simulink model "min_cost_function_and_vopt_FCS_MPC_6Phase_PMSM"  (R2022a)
settings: Solver=FixedStepDiscrete  StartTime=0.0  StopTime=10.0  RelTol=1e-3
values from neighbouring files (symbols this model uses):
  f_c = 100000    [MPC_params.m]
libraries: hdlsllib x2
settings Model: DataTypeOverride=Off  Creator=Andre Merx  LastModifiedBy=Andre Merx
settings SolverCC: AlgebraicLoopSolver=TrustRegion
settings DataIOCC: LimitDataPoints=on  SaveOutput=off  SaveTime=off
settings OptimizationCC: BlockReduction=off  ConditionallyExecuteInputs=off  DefaultParameterBehavior=Inlined  LifeSpan=inf
settings DebuggingCC: AlgebraicLoopMsg=error  SingleTaskRateTransMsg=error  UnconnectedInputMsg=warning  UnconnectedOutputMsg=warning  UnconnectedLineMsg=warning  AllowSymbolicDim=off  StrictBusMsg=ErrorOnBusTreatedAsVector  SFUnexpectedBacktrackingDiag=warning  SFNoUnconditionalDefaultTransitionDiag=warning  SFExecutionAtInitializationDiag=none  SFMachineParentedDataDiag=warning  ArithmeticOperatorsInVariantConditions=warning
settings HardwareCC: ProdBitPerPointer=32  ProdBitPerSizeT=32  ProdBitPerPtrDiffT=32  ProdLargestAtomicFloat=None  ProdIntDivRoundTo=Undefined  ProdEndianess=Unspecified  ProdWordSize=32  ProdHWDeviceType=ASIC/FPGA->ASIC/FPGA  ProdEqTarget=off
settings SFSimCC: SimUseLocalCustomCode=off  CustomCodeUndefinedFunction=UseInterfaceOnly
settings RTWCC: RTWUseLocalCustomCode=off
settings CodeAppCC: StateflowObjectComments=on
settings GRTTargetCC: TargetLangStandard=C89/C90 (ANSI)
settings ConfigComp: CovScope=ReferencedModels  CovMetricSettings=dw  CovSaveCumulativeToWorkspaceVar=on  CovSaveSingleToWorkspaceVar=on  CovExternalEMLEnable=off  CovSFcnEnable=off

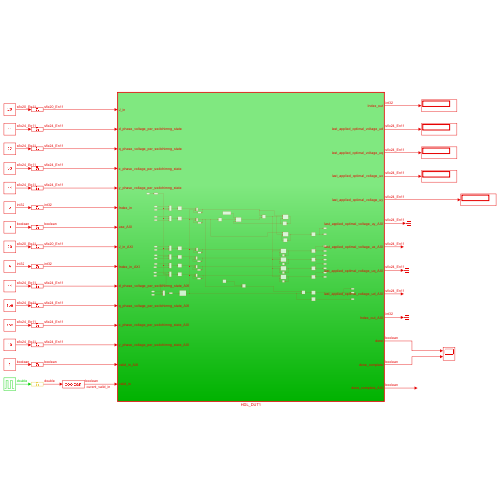
[thumbnail: Simulink's stored preview of the top-level diagram]
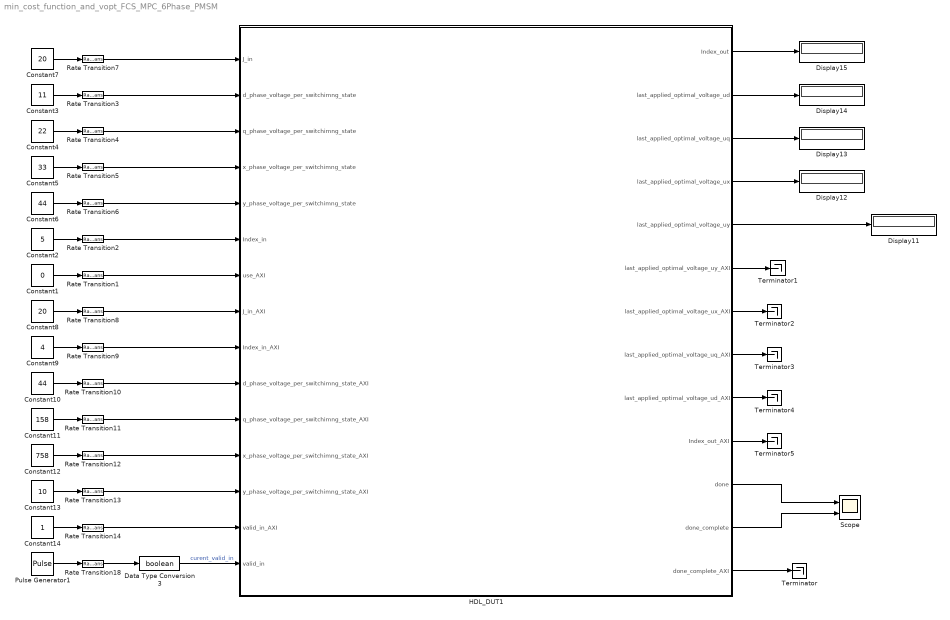
== system min_cost_function_and_vopt_FCS_MPC_6Phase_PMSM ==
  Constant1 : Constant  Value=0  OutDataTypeStr=boolean  SampleTime=-1
  Constant10 : Constant  Value=44  OutDataTypeStr=fixdt(1,24,11)  SampleTime=-1  LockScale=on
  Constant11 : Constant  Value=158  OutDataTypeStr=fixdt(1,24,11)  SampleTime=-1
  Constant12 : Constant  Value=758  OutDataTypeStr=fixdt(1,24,11)  SampleTime=-1
  Constant13 : Constant  Value=10  OutDataTypeStr=fixdt(1,24,11)  SampleTime=-1
  Constant14 : Constant  OutDataTypeStr=boolean  SampleTime=-1
  Constant2 : Constant  Value=5  OutDataTypeStr=int32  SampleTime=-1
  Constant3 : Constant  Value=11  OutDataTypeStr=fixdt(1,24,11)  SampleTime=-1  LockScale=on
  Constant4 : Constant  Value=22  OutDataTypeStr=fixdt(1,24,11)  SampleTime=-1
  Constant5 : Constant  Value=33  OutDataTypeStr=fixdt(1,24,11)  SampleTime=-1
  Constant6 : Constant  Value=44  OutDataTypeStr=fixdt(1,24,11)  SampleTime=-1
  Constant7 : Constant  Value=20  OutDataTypeStr=fixdt(1,20,11)  SampleTime=-1
  Constant8 : Constant  Value=20  OutDataTypeStr=fixdt(1,20,11)  SampleTime=-1
  Constant9 : Constant  Value=4  OutDataTypeStr=int32  SampleTime=-1
  Data Type Conversion3 : DataTypeConversion  OutDataTypeStr=boolean  SaturateOnIntegerOverflow=off  RndMeth=Floor
  Display{11..15} (5 alike) : Display
  HDL_DUT1 : Subsystem  TreatAsAtomicUnit=on
  Pulse Generator1 : DiscretePulseGenerator  PulseType=Time based  Period=1/f_c
  Rate Transition{1..14,18} (15 alike) : RateTransition  OutPortSampleTime=Rt
  Scope : Scope  NumInputPorts=2
  Terminator{,1..5} (6 alike) : Terminator
  wires:
  Data Type Conversion3/1 -> HDL_DUT1/15(valid_in)  "curent_valid_in"
  Pulse Generator1/1 -> Rate Transition18/1
  Rate Transition18/1 -> Data Type Conversion3/1
  Constant2/1 -> Rate Transition2/1
  Rate Transition2/1 -> HDL_DUT1/6(Index_in)
  HDL_DUT1/5(last_applied_optimal_voltage_uy) -> Display11/1
  HDL_DUT1/4(last_applied_optimal_voltage_ux) -> Display12/1
  HDL_DUT1/3(last_applied_optimal_voltage_uq) -> Display13/1
  HDL_DUT1/2(last_applied_optimal_voltage_ud) -> Display14/1
  HDL_DUT1/1(Index_out) -> Display15/1
  Constant3/1 -> Rate Transition3/1
  Rate Transition3/1 -> HDL_DUT1/2(d_phase_voltage_per_switchimng_state)
  Constant4/1 -> Rate Transition4/1
  Rate Transition4/1 -> HDL_DUT1/3(q_phase_voltage_per_switchimng_state)
  Constant5/1 -> Rate Transition5/1
  Rate Transition5/1 -> HDL_DUT1/4(x_phase_voltage_per_switchimng_state)
  Constant6/1 -> Rate Transition6/1
  Rate Transition6/1 -> HDL_DUT1/5(y_phase_voltage_per_switchimng_state)
  Constant7/1 -> Rate Transition7/1
  Rate Transition7/1 -> HDL_DUT1/1(J_in)
  HDL_DUT1/13(done_complete_AXI) -> Terminator/1
  HDL_DUT1/6(last_applied_optimal_voltage_uy_AXI) -> Terminator1/1
  HDL_DUT1/7(last_applied_optimal_voltage_ux_AXI) -> Terminator2/1
  HDL_DUT1/8(last_applied_optimal_voltage_uq_AXI) -> Terminator3/1
  HDL_DUT1/9(last_applied_optimal_voltage_ud_AXI) -> Terminator4/1
  HDL_DUT1/10(Index_out_AXI) -> Terminator5/1
  Constant1/1 -> Rate Transition1/1
  Rate Transition1/1 -> HDL_DUT1/7(use_AXI)
  Constant8/1 -> Rate Transition8/1
  Rate Transition8/1 -> HDL_DUT1/8(J_in_AXI)
  Constant9/1 -> Rate Transition9/1
  Rate Transition9/1 -> HDL_DUT1/9(Index_in_AXI)
  Rate Transition12/1 -> HDL_DUT1/12(x_phase_voltage_per_switchimng_state_AXI)
  Constant11/1 -> Rate Transition11/1
  Constant12/1 -> Rate Transition12/1
  Constant13/1 -> Rate Transition13/1
  Rate Transition13/1 -> HDL_DUT1/13(y_phase_voltage_per_switchimng_state_AXI)
  Constant10/1 -> Rate Transition10/1
  Rate Transition11/1 -> HDL_DUT1/11(q_phase_voltage_per_switchimng_state_AXI)
  Rate Transition10/1 -> HDL_DUT1/10(d_phase_voltage_per_switchimng_state_AXI)
  Constant14/1 -> Rate Transition14/1
  Rate Transition14/1 -> HDL_DUT1/14(valid_in_AXI)
  HDL_DUT1/11(done) -> Scope/1
  HDL_DUT1/12(done_complete) -> Scope/2

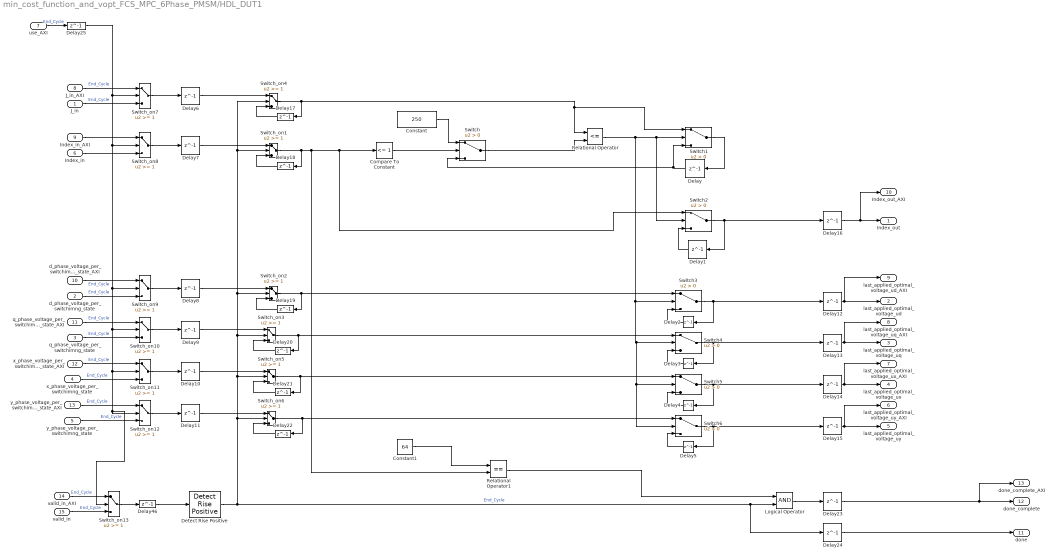
== system min_cost_function_and_vopt_FCS_MPC_6Phase_PMSM/HDL_DUT1 ==
  J_in : Inport
  d_phase_voltage_per_switchimng_state : Inport  Port=2
  q_phase_voltage_per_switchimng_state : Inport  Port=3
  x_phase_voltage_per_switchimng_state : Inport  Port=4
  y_phase_voltage_per_switchimng_state : Inport  Port=5
  Index_in : Inport  Port=6
  use_AXI : Inport  Port=7
  J_in_AXI : Inport  Port=8
  Index_in_AXI : Inport  Port=9
  d_phase_voltage_per_switchimng_state_AXI : Inport  Port=10
  q_phase_voltage_per_switchimng_state_AXI : Inport  Port=11
  x_phase_voltage_per_switchimng_state_AXI : Inport  Port=12
  y_phase_voltage_per_switchimng_state_AXI : Inport  Port=13
  valid_in_AXI : Inport  Port=14
  valid_in : Inport  Port=15
  Compare To Constant : hdlsllib/Logic and Bit Operations/Compare To Constant  relop=<=  const=1  OutDataTypeStr=boolean
      settings: SourceProductBaseCode=SL
  Constant : Constant  Value=250  OutDataTypeStr=fixdt(1,20,11)  SampleTime=-1
  Constant1 : Constant  Value=64  OutDataTypeStr=int32  SampleTime=-1
  Delay{,1..25,46} (27 alike) : Delay  DelayLength=1
  Detect Rise Positive : hdlsllib/Logic and Bit Operations/Detect Rise Positive  vinit=0  OutDataTypeStr=boolean
      settings: SourceProductBaseCode=SL
  Logical Operator : Logic  AllPortsSameDT=off  OutDataTypeStr=boolean
  Relational Operator : RelationalOperator  Operator=<=  OutDataTypeStr=boolean  RndMeth=Simplest  InputSameDT=off
  Relational Operator1 : RelationalOperator  Operator===  OutDataTypeStr=boolean  RndMeth=Simplest  InputSameDT=off
  Switch{,1..6} (7 alike) : Switch  Criteria=u2 > Threshold  SaturateOnIntegerOverflow=off  InputSameDT=off
  Switch_on{1..13} (13 alike) : Switch  Threshold=1  OutDataTypeStr=Inherit: Inherit via back propagation  RndMeth=Simplest  SaturateOnIntegerOverflow=off  InputSameDT=off
  Index_out : Outport
  last_applied_optimal_voltage_ud : Outport  Port=2
  last_applied_optimal_voltage_uq : Outport  Port=3
  last_applied_optimal_voltage_ux : Outport  Port=4
  last_applied_optimal_voltage_uy : Outport  Port=5
  last_applied_optimal_voltage_uy_AXI : Outport  Port=6
  last_applied_optimal_voltage_ux_AXI : Outport  Port=7
  last_applied_optimal_voltage_uq_AXI : Outport  Port=8
  last_applied_optimal_voltage_ud_AXI : Outport  Port=9
  Index_out_AXI : Outport  Port=10
  done : Outport  Port=11
  done_complete : Outport  Port=12
  done_complete_AXI : Outport  Port=13
  wires:
  J_in/1 -> Switch_on7/3  "End_Cycle"
  d_phase_voltage_per_switchimng_state/1 -> Switch_on9/3  "End_Cycle"
  y_phase_voltage_per_switchimng_state/1 -> Switch_on12/3  "End_Cycle"
  x_phase_voltage_per_switchimng_state/1 -> Switch_on11/3  "End_Cycle"
  q_phase_voltage_per_switchimng_state/1 -> Switch_on10/3  "End_Cycle"
  Switch5/1 -> Delay14/1, Delay4/1
  Delay3/1 -> Switch4/3
  Relational Operator/1 -> Switch5/2, Switch6/2, Switch4/2, Switch3/2, Switch2/2, Switch1/2
  Compare To Constant/1 -> Switch/2
  Switch1/1 -> Delay/1
  Switch6/1 -> Delay15/1, Delay5/1
  Delay4/1 -> Switch5/3
  Switch4/1 -> Delay13/1, Delay3/1
  Index_in/1 -> Switch_on8/3
  Switch/1 -> Relational Operator/2
  Switch2/1 -> Delay16/1, Delay1/1
  Delay1/1 -> Switch2/3
  Delay5/1 -> Switch6/3
  Delay/1 -> Switch/3, Switch1/3
  Switch3/1 -> Delay12/1, Delay2/1
  Delay2/1 -> Switch3/3
  Constant/1 -> Switch/1
  Switch_on4/1 -> Relational Operator/1, Switch1/1, Delay17/1
  Switch_on1/1 -> Delay18/1, Relational Operator1/2, Switch2/1, Compare To Constant/1
  Switch_on2/1 -> Delay19/1, Switch3/1
  Switch_on3/1 -> Delay20/1, Switch4/1
  Switch_on5/1 -> Switch5/1, Delay21/1
  Switch_on6/1 -> Switch6/1, Delay22/1
  Delay12/1 -> last_applied_optimal_voltage_ud_AXI/1, last_applied_optimal_voltage_ud/1
  Delay13/1 -> last_applied_optimal_voltage_uq_AXI/1, last_applied_optimal_voltage_uq/1
  Delay15/1 -> last_applied_optimal_voltage_uy_AXI/1, last_applied_optimal_voltage_uy/1
  Delay16/1 -> Index_out_AXI/1, Index_out/1
  Delay46/1 -> Detect Rise Positive/1
  valid_in/1 -> Switch_on13/3  "End_Cycle"
  Detect Rise Positive/1 -> Switch_on4/2, Switch_on1/2, Switch_on2/2, Switch_on3/2, Switch_on5/2, Switch_on6/2, Delay24/1, Logical Operator/2  "End_Cycle"
  Delay6/1 -> Switch_on4/1
  Delay17/1 -> Switch_on4/3
  Delay7/1 -> Switch_on1/1
  Delay18/1 -> Switch_on1/3
  Delay8/1 -> Switch_on2/1
  Delay19/1 -> Switch_on2/3
  Delay9/1 -> Switch_on3/1
  Delay20/1 -> Switch_on3/3
  Delay10/1 -> Switch_on5/1
  Delay21/1 -> Switch_on5/3
  Delay11/1 -> Switch_on6/1
  Delay22/1 -> Switch_on6/3
  Delay23/1 -> done_complete_AXI/1, done_complete/1
  Logical Operator/1 -> Delay23/1
  Relational Operator1/1 -> Logical Operator/1
  Delay24/1 -> done/1
  Constant1/1 -> Relational Operator1/1
  Switch_on7/1 -> Delay6/1
  J_in_AXI/1 -> Switch_on7/1  "End_Cycle"
  Switch_on8/1 -> Delay7/1
  Index_in_AXI/1 -> Switch_on8/1
  Switch_on9/1 -> Delay8/1
  d_phase_voltage_per_switchimng_state_AXI/1 -> Switch_on9/1  "End_Cycle"
  Switch_on10/1 -> Delay9/1
  q_phase_voltage_per_switchimng_state_AXI/1 -> Switch_on10/1  "End_Cycle"
  Switch_on11/1 -> Delay10/1
  x_phase_voltage_per_switchimng_state_AXI/1 -> Switch_on11/1  "End_Cycle"
  Switch_on12/1 -> Delay11/1
  y_phase_voltage_per_switchimng_state_AXI/1 -> Switch_on12/1  "End_Cycle"
  Switch_on13/1 -> Delay46/1
  valid_in_AXI/1 -> Switch_on13/1  "End_Cycle"
  Delay14/1 -> last_applied_optimal_voltage_ux_AXI/1, last_applied_optimal_voltage_ux/1
  use_AXI/1 -> Delay25/1  "End_Cycle"
  Delay25/1 -> Switch_on9/2, Switch_on10/2, Switch_on11/2, Switch_on13/2, Switch_on12/2, Switch_on8/2, Switch_on7/2
